simulink model "app03_1_capture_camera"  (R2016a)
settings: Solver=FixedStepAuto  StartTime=0.0  StopTime=10.0  RelTol=1e-3
libraries: embdlinuxlib x2, simulink x1
settings Model: SimulationMode=external  Creator=ohori  LastModifiedBy=ohori
settings SolverCC: PositivePriorityOrder=on
settings OptimizationCC: OptimizeModelRefInitCode=on  LifeSpan=1  MaxStackSize=64
settings HardwareCC: ProdBitPerPointer=32  ProdLargestAtomicInteger=Long  ProdLargestAtomicFloat=Double  ProdWordSize=32  ProdHWDeviceType=ARM Compatible->ARM Cortex  UseEmbeddedCoderFeatures=off  UseSimulinkCoderFeatures=off
settings RTWCC: SystemTargetFile=ert.tlc  HardwareBoard=Raspberry Pi  TemplateMakefile=ert_default_tmf  RTWVerbose=off  Toolchain=GNU GCC Raspberry Pi  IncludeHyperlinkInReport=on
settings CodeAppCC: ForceParamTrailComments=on  OperatorAnnotations=on  SimulinkDataObjDesc=on  SFDataObjDesc=on  MATLABFcnDesc=on  MangleLength=10  InsertBlockDesc=on  MATLABSourceComments=on
settings ERTTargetCC: SupportNonInlinedSFcns=on  SupportVariableSizeSignals=on  ExtMode=on  ExtModeMexArgs='169.254.0.2' 0 17725  ERTSrcFileBannerTemplate=codertarget_code_template.cgt  ERTHdrFileBannerTemplate=codertarget_code_template.cgt  ERTDataSrcFileTemplate=codertarget_code_template.cgt  ERTDataHdrFileTemplate=codertarget_code_template.cgt

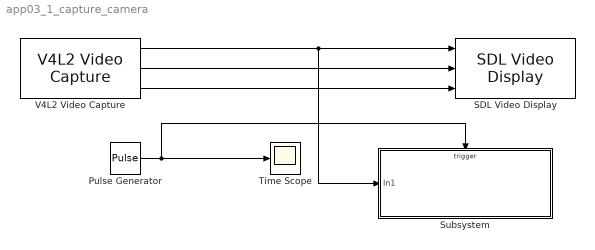
== system app03_1_capture_camera ==
  Pulse Generator : DiscretePulseGenerator  Period=10  SampleTime=0.1
  SDL Video Display : embdlinuxlib/SDL Video Display  pixelFormat=YCbCr 4:2:2  pixelOrder=Planar  rowMajor=on  blockPlatform=Raspberry Pi
  Subsystem : Subsystem
  Time Scope : Scope
  V4L2 Video Capture : embdlinuxlib/V4L2 Video Capture  m_devName='/dev/video0'  roi=[0, 0, 640, 480]  imSizeSelection=320x240  imSize=[640, 480]  pixelFormat=YCbCr 4:2:2  pixelOrder=Planar  sampleTime=1/10  simOutput=Colorbars  blockPlatform=Raspberry Pi
  wires:
  V4L2 Video Capture/1 -> Subsystem/1(In1), SDL Video Display/1
  V4L2 Video Capture/2 -> SDL Video Display/2
  V4L2 Video Capture/3 -> SDL Video Display/3
  Pulse Generator/1 -> Time Scope/1, Subsystem/Trigger

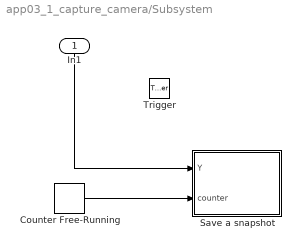
== system app03_1_capture_camera/Subsystem ==
  In1 : Inport
  Trigger : TriggerPort  VariantControl=Variant
  Counter Free-Running : simulink/Sources/Counter Free-Running  NumBits=32  tsamp=-1
  Save a snapshot : MATLAB Function  TreatAsAtomicUnit=on
  wires:
  In1/1 -> Save a snapshot/1(Y)
  Counter Free-Running/1 -> Save a snapshot/2(counter)

== matlab function app03_1_capture_camera/Subsystem/Save a snapshot ==
  data: Y input; counter input
function fcn(Y, counter)
%#codegen

% Save 160x120 grayscale image to a file
format = ['%d ', 0];
fname  = coder.nullcopy(uint8(zeros(1, 32)));
coder.ceval('sprintf', coder.wref(fname), ['img%d.dat', 0], counter);
fd = coder.opaque('FILE *');
fd = coder.ceval('fopen', fname, ['w', 0]);
for i = 1:160
    for j = 1:120
        coder.ceval('fprintf', fd, format, Y(i, j));
    end
end
coder.ceval('fclose', fd);
